simulink model "d_analog_komp_R2018b"  (R2018b)
settings: Solver=VariableStepAuto  StartTime=0.0  StopTime=10.0  MaxStep=0.00001  RelTol=1e-3
undefined symbols (not defined in the file): Kd, Kda, Kp, Kpa, st, T0, T1
settings Model: Creator=bedla  LastModifiedBy=bedla

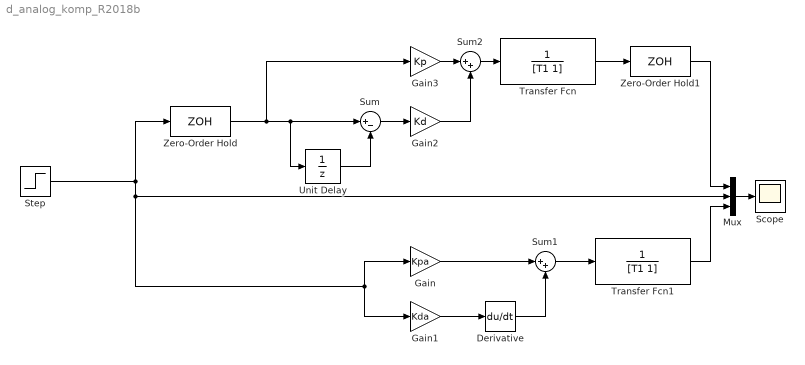
== system d_analog_komp_R2018b ==
  Derivative : Derivative
  Gain : Gain  Gain=Kpa
  Gain1 : Gain  Gain=Kda
  Gain2 : Gain  Gain=Kd
  Gain3 : Gain  Gain=Kp
  Mux : Mux  Inputs=3
  Scope : Scope
  Step : Step  After=st  SampleTime=0
  Sum : Sum  Inputs=|+-
  Sum1 : Sum  Inputs=|++
  Sum2 : Sum  Inputs=|++
  Transfer Fcn : TransferFcn  Denominator=[T1 1]
  Transfer Fcn1 : TransferFcn  Denominator=[T1 1]
  Unit Delay : UnitDelay  SampleTime=T0  HasFrameUpgradeWarning=on
  Zero-Order Hold : ZeroOrderHold  SampleTime=T0
  Zero-Order Hold1 : ZeroOrderHold  SampleTime=T0
  wires:
  Step/1 -> Mux/2, Gain/1, Gain1/1, Zero-Order Hold/1
  Gain1/1 -> Derivative/1
  Gain/1 -> Sum1/1
  Derivative/1 -> Sum1/2
  Sum1/1 -> Transfer Fcn1/1
  Gain2/1 -> Sum2/2
  Zero-Order Hold/1 -> Gain3/1, Sum/1, Unit Delay/1
  Sum/1 -> Gain2/1
  Unit Delay/1 -> Sum/2
  Gain3/1 -> Sum2/1
  Mux/1 -> Scope/1
  Sum2/1 -> Transfer Fcn/1
  Transfer Fcn/1 -> Zero-Order Hold1/1
  Transfer Fcn1/1 -> Mux/3
  Zero-Order Hold1/1 -> Mux/1
